simulink model "system_dyninv_2nd_order"  (R2018b)
settings: Solver=ode8  StartTime=0.0  StopTime=10  FixedStep=0.01  RelTol=1e-3
values from neighbouring files (symbols this model uses):
  A = [0 1; -w^2 -2*z*w]    [dyninv_2nd_order.m]
  B = [0; w^2]    [dyninv_2nd_order.m]
  C = [1 0; 0 1]    [dyninv_2nd_order.m]
  CA = [0 1]*A    [dyninv_2nd_order.m]
  invCB = inv([0 1]*B)    [dyninv_2nd_order.m]
  K1 = 4    [dyninv_2nd_order.m]
  K2 = 1    [dyninv_2nd_order.m]
settings Model: Creator=suvo.ganguli  LastModifiedBy=suvo.ganguli

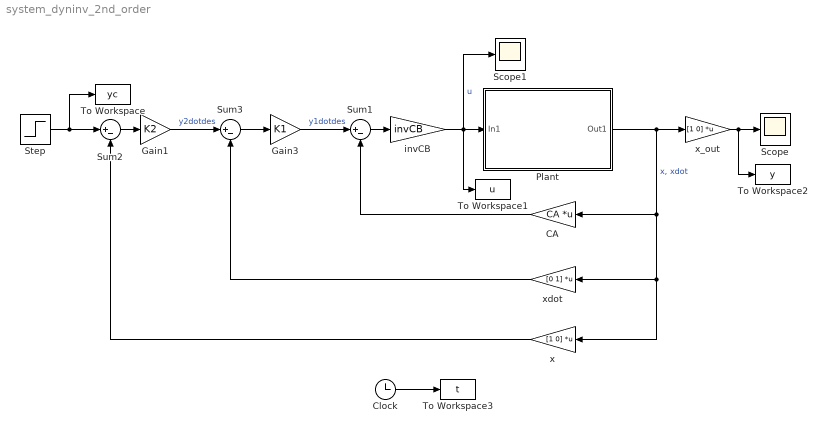
== system system_dyninv_2nd_order ==
  CA : Gain  Gain=CA  Multiplication=Matrix(K*u)
  Clock : Clock
  Gain1 : Gain  Gain=K2
  Gain3 : Gain  Gain=K1
  Plant : Subsystem
  Scope : Scope
  Scope1 : Scope
  Step : Step  SampleTime=0
  Sum1 : Sum  Inputs=|+-
  Sum2 : Sum  Inputs=|+-
  Sum3 : Sum  Inputs=|+-
  To Workspace : ToWorkspace  VariableName=yc  SampleTime=-1
  To Workspace1 : ToWorkspace  VariableName=u  SampleTime=-1
  To Workspace2 : ToWorkspace  VariableName=y  SampleTime=-1
  To Workspace3 : ToWorkspace  VariableName=t  SampleTime=-1
  invCB : Gain  Gain=invCB
  x : Gain  Gain=[1 0]  Multiplication=Matrix(K*u)
  x_out : Gain  Gain=[1 0]  Multiplication=Matrix(K*u)
  xdot : Gain  Gain=[0 1]  Multiplication=Matrix(K*u)
  wires:
  Plant/1(Out1) -> x_out/1, x/1, xdot/1, CA/1  "x, xdot"
  xdot/1 -> Sum3/2
  CA/1 -> Sum1/2
  Sum2/1 -> Gain1/1
  x/1 -> Sum2/2
  x_out/1 -> To Workspace2/1, Scope/1
  Sum3/1 -> Gain3/1
  Step/1 -> To Workspace/1, Sum2/1
  Sum1/1 -> invCB/1
  invCB/1 -> To Workspace1/1, Plant/1(In1), Scope1/1  "u"
  Gain3/1 -> Sum1/1  "y1dotdes"
  Gain1/1 -> Sum3/1  "y2dotdes"
  Clock/1 -> To Workspace3/1

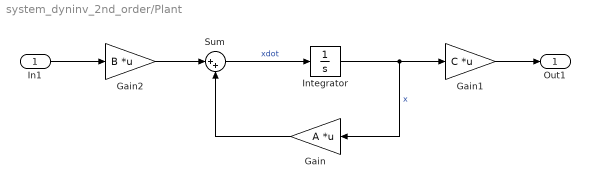
== system system_dyninv_2nd_order/Plant ==
  In1 : Inport
  Gain : Gain  Gain=A  Multiplication=Matrix(K*u)
  Gain1 : Gain  Gain=C  Multiplication=Matrix(K*u)
  Gain2 : Gain  Gain=B  Multiplication=Matrix(K*u)
  Integrator : Integrator
  Sum : Sum  Inputs=|++
  Out1 : Outport
  wires:
  Integrator/1 -> Gain1/1, Gain/1  "x"
  Sum/1 -> Integrator/1  "xdot"
  Gain/1 -> Sum/2
  In1/1 -> Gain2/1
  Gain2/1 -> Sum/1
  Gain1/1 -> Out1/1
